simulink model "TempControlExperimentTest"  (R2016b)
settings: Solver=FixedStepDiscrete  StartTime=0.0  StopTime=inf  FixedStep=1  RelTol=1e-3  EnableMultiTasking=on
libraries: EEE481Arduino x4
settings Model: ExtModeTrigDuration=2  Creator=rsjoshi1  LastModifiedBy=rsjoshi1
settings OptimizationCC: LifeSpan=Inf  MaxStackSize=64
settings DebuggingCC: SFUnexpectedBacktrackingDiag=warning  SFNoUnconditionalDefaultTransitionDiag=warning  SFExecutionAtInitializationDiag=none
settings HardwareCC: ProdBitPerPointer=32  ProdBitPerSizeT=32  ProdBitPerPtrDiffT=32  ProdLargestAtomicInteger=Long  ProdLargestAtomicFloat=Double  ProdWordSize=32  ProdHWDeviceType=ARM Compatible->ARM Cortex
settings RTWCC: SystemTargetFile=ert.tlc  HardwareBoard=Arduino Due  TLCOptions=-aInlineSetEventsForThisBaseRateFcn=TLC_FALSE -aSuppressMultiTaskScheduler=TLC_FALSE -aRateBasedStepFcn=1  TemplateMakefile=ert_default_tmf  Description=Embedded Coder  GenerateReport=on  Toolchain=Arduino ARM v1.6.7  BuildConfiguration=Faster Runs  IncludeHyperlinkInReport=on  LaunchReport=on  GenerateTraceInfo=on  GenerateTraceReport=on  GenerateTraceReportSl=on  GenerateTraceReportSf=on  GenerateTraceReportEml=on
settings CodeAppCC: ForceParamTrailComments=on  IgnoreCustomStorageClasses=off  OperatorAnnotations=on  SimulinkDataObjDesc=on  SFDataObjDesc=on  MATLABFcnDesc=on  InsertBlockDesc=on  MATLABSourceComments=on
settings ERTTargetCC: SupportContinuousTime=on  SupportVariableSizeSignals=on
settings ConfigComp: CovMetricSettings=dw  CovHtmlReporting=on  CovSaveCumulativeToWorkspaceVar=on  CovSaveSingleToWorkspaceVar=on  CovExternalEMLEnable=off

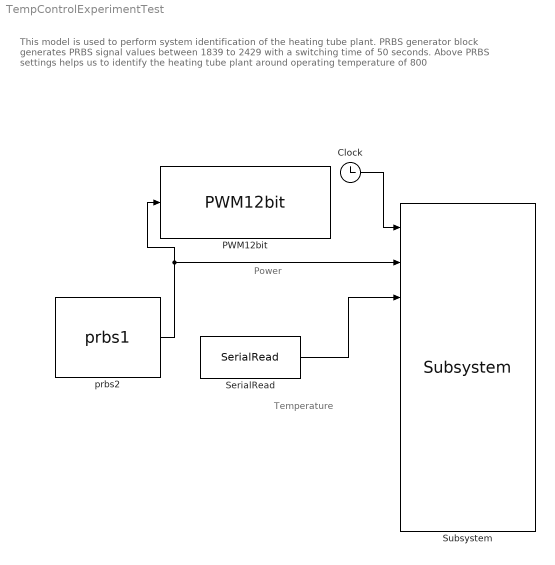
== system TempControlExperimentTest ==
  note: Power
  note: Temperature
  note: This model is used to perform system identification of the heating tube plant.
      | PRBS generator block generates PRBS signal values between 1839 to 2429 with a switching time of 50 seconds.
      | Above PRBS settings helps us to identify the heating tube plant around operating temperature of 800
  Clock : Clock
  PWM12bit : EEE481Arduino/PWM12bit  PwmPort=2  Tsa=0
  SerialRead : EEE481Arduino/SerialRead  serialNum=2  Ts=-1
  Subsystem : EEE481Arduino/Subsystem  Tsa=1  rate=0  per=0
  prbs2 : EEE481Arduino/prbs1  Tsa=Tsa  Tsw=50  Lz=400  Lv=300  Nc=1  initLevel=4095*0.52
  wires:
  prbs2/1 -> PWM12bit/1, Subsystem/2
  SerialRead/1 -> Subsystem/3
  Clock/1 -> Subsystem/1
